simulink library "rtwdemowidgets"  (Simulink 6.0)
settings: Solver=ode45  SolverMode=SingleTasking  StartTime=0.0  StopTime=10.0  RelTol=1e-3
settings Model: Creator=The MathWorks Inc.  LastModifiedBy=batserve  ExtModeAutoUpdateStatusClock=off
settings DataIOCC: SignalLoggingName=logsOut
settings OptimizationCC: BooleanDataType=off
settings DebuggingCC: CheckExecutionContextPreStartOutputMsg=on  CheckExecutionContextRuntimeOutputMsg=on  SolverPrmCheckMsg=none
settings HardwareCC: TargetUnknown=on
settings ModelReferenceCC: UpdateModelReferenceTargets=IfOutOfDate

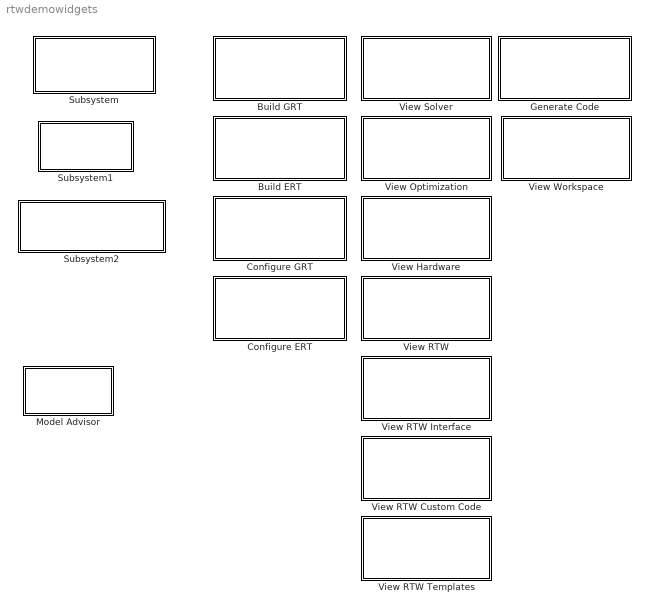
== system rtwdemowidgets ==
  Build ERT : Subsystem  PropExecContextAcrossSSBoundary=on  mask{attrib_overrides={}}
      mask prompts: attrib_overrides "List of attributes to preserve (cell of strings):"
      mask help: Enter the attributes of the configuration set that you want preserved. Otherwise, the default configuration script will override your current settings.
      settings: OpenFcn=|
      | model=bdroot;
      |                   overrides=get_param(gcb,'attrib_overrides');
      | try
      |   rtwconfiguredemo(model,'noop',false,overrides);
      |   rtwbuilddemomodel(model);
      | catch
      |   error(lasterr);
      | end
      mask Display:
      | disp(['Generate Code Using\n',...
      | 	  'Real-Time Workshop\n',...
      | 	  'Embedded Coder\n'...
      | 	  '(double-click)'])
  Build GRT : Subsystem  PropExecContextAcrossSSBoundary=on  mask{attrib_overrides={}}
      mask prompts: attrib_overrides "List of attributes to preserve (cell of strings):"
      mask help: Enter the attributes of the configuration set that you want preserved. Otherwise, the default configuration script will override your current settings.
      settings: OpenFcn=|
      | model=bdroot;
      |                   overrides=get_param(gcb,'attrib_overrides');
      | try
      |   rtwconfiguredemo(model,'noop',true,overrides);
      |   rtwbuilddemomodel(model);
      | catch
      |   error(lasterr);
      | end
      mask Display:
      | disp(['Generate Code Using\n',...
      | 	  'Real-Time Workshop\n',...
      | 	  '(double-click)'])
  Configure ERT : Subsystem  PropExecContextAcrossSSBoundary=on
      settings: OpenFcn=|
      | model=bdroot;
      | try
      |   rtwconfiguredemo(model,'noop',false,{});
      | catch
      |   error(lasterr);
      | end
      mask Display:
      | disp(['Configure for\n',...
      | 	  'Real-Time Workshop\n',...
      | 	  'Embedded Coder\n',...
      | 	  '(double-click)'])
  Configure GRT : Subsystem  PropExecContextAcrossSSBoundary=on
      settings: OpenFcn=|
      | model=bdroot;
      | try
      |   rtwconfiguredemo(model,'noop',true,{});
      | catch
      |   error(lasterr);
      | end
      mask Display:
      | disp(['Configure for\n',...
      | 	  'Real-Time Workshop\n',...
      | 	  '(double-click)'])
  Generate Code : Subsystem  PropExecContextAcrossSSBoundary=on
      settings: OpenFcn=|
      | model=bdroot;
      | try
      |   rtwbuilddemomodel(model);
      | catch
      |   error(lasterr);
      | end
      mask Display:
      | disp(['Generate Code\n',...
      | 	  '(double-click)'])
  Model Advisor : Subsystem  PropExecContextAcrossSSBoundary=on  mask{attrib_overrides={}}
      mask prompts: attrib_overrides "List of attributes to preserve (cell of strings):"
      mask help: Enter the attributes of the configuration set that you want preserved. Otherwise, the default configuration script will override your current settings.
      settings: OpenFcn=modeladvisor(bdroot);
      mask Display:
      | text(.05,.5,['Launch Model\n',...
      | 	  'Advisor ..','.'])
  Subsystem : Subsystem  PropExecContextAcrossSSBoundary=on
      settings: OpenFcn=rtwbuilddemomodel(bdroot);
      mask Display: disp('Generate Code\n(double-click)')
  Subsystem1 : Subsystem  AncestorBlock=rtwdemowidgets/Subsystem  PropExecContextAcrossSSBoundary=on
      settings: OpenFcn=rtwbuilddemomodel(bdroot);
      mask Display: disp('Generate\nCode')
  Subsystem2 : Subsystem  PropExecContextAcrossSSBoundary=on
      settings: OpenFcn=disp('');
      mask Display:
      | text(0,.5,sprintf([...
      | 		'Model is configured for ERT\n',...
      | 		'code generation.  Will default\n', ...
      | 		'to GRT if Real-Time Workshop\n', ...
      | 		'Embedded Coder is not installed.',...
      | 	]));
  View Hardware : Subsystem  PropExecContextAcrossSSBoundary=on
      settings: OpenFcn=|
      | slCfgPrmDlg(bdroot,'Open');
      | slCfgPrmDlg(bdroot,'TurnToPage','Hardware Implementation');
      mask Display: disp('View Hardware\nConfiguration\n(double-click)')
  View Optimization : Subsystem  PropExecContextAcrossSSBoundary=on
      settings: OpenFcn=|
      | model = bdroot;
      | slCfgPrmDlg(model,'Open');
      | slCfgPrmDlg(bdroot,'TurnToPage','Optimization');
      mask Display: disp('View Optimization\nConfiguration\n(double-click)')
  View RTW : Subsystem  PropExecContextAcrossSSBoundary=on
      settings: OpenFcn=|
      | slCfgPrmDlg(bdroot,'Open');
      | slCfgPrmDlg(bdroot,'TurnToPage','Real-Time Workshop');
      mask Display: disp('View Real-\nTime Workshop\nConfiguration\n(double-click)')
  View RTW Custom Code : Subsystem  PropExecContextAcrossSSBoundary=on
      settings: OpenFcn=|
      | slCfgPrmDlg(bdroot,'Open');
      | slCfgPrmDlg(bdroot,'TurnToPage','Real-Time Workshop/Custom Code');
      mask Display: disp('View Custom Code\nConfiguration\n(double-click)')
  View RTW Interface : Subsystem  PropExecContextAcrossSSBoundary=on
      settings: OpenFcn=|
      | slCfgPrmDlg(bdroot,'Open');
      | slCfgPrmDlg(bdroot,'TurnToPage','Real-Time Workshop/Interface');
      mask Display: disp('View Interface\nConfiguration\n(double-click)')
  View RTW Templates : Subsystem  PropExecContextAcrossSSBoundary=on
      settings: OpenFcn=|
      | slCfgPrmDlg(bdroot,'Open');
      | slCfgPrmDlg(bdroot,'TurnToPage','Real-Time Workshop/Templates');
      mask Display: disp('View Templates\nConfiguration\n(double-click)')
  View Solver : Subsystem  PropExecContextAcrossSSBoundary=on
      settings: OpenFcn=|
      | slCfgPrmDlg(bdroot,'Open');
      | slCfgPrmDlg(bdroot,'TurnToPage','Solver');
      mask Display: disp('View Solver\nConfiguration\n(double-click)')
  View Workspace : Subsystem  PropExecContextAcrossSSBoundary=on
      settings: OpenFcn=rtwprivate daexplrwsview;
      mask Display: disp('View Workspace\nVariables\n(double-click)')

== system rtwdemowidgets/Build ERT ==

== system rtwdemowidgets/Build GRT ==

== system rtwdemowidgets/Configure ERT ==

== system rtwdemowidgets/Configure GRT ==

== system rtwdemowidgets/Generate Code ==

== system rtwdemowidgets/Model Advisor ==

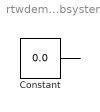
== system rtwdemowidgets/Subsystem ==
  Constant : Constant  Value=0.0  OutDataTypeMode=Specify via dialog  ConRadixGroup=Best Precision: Vector-wise  OutScaling=2^-1000
  wires:
  Constant/1 -> ?

== system rtwdemowidgets/Subsystem1 ==

== system rtwdemowidgets/Subsystem2 ==

== system rtwdemowidgets/View Hardware ==

== system rtwdemowidgets/View Optimization ==

== system rtwdemowidgets/View RTW ==

== system rtwdemowidgets/View RTW Custom Code ==

== system rtwdemowidgets/View RTW Interface ==

== system rtwdemowidgets/View RTW Templates ==

== system rtwdemowidgets/View Solver ==

== system rtwdemowidgets/View Workspace ==
